simulink model "IP"  (Simulink 5.0)
settings: Solver=ode5  SolverMode=SingleTasking  StartTime=0.0  StopTime=inf  FixedStep=0.001  RelTol=1e-3
libraries: pci1711 x3
settings Model: LastModifiedBy=AD  ExtModeMexFile=rtwinext  SimulationMode=external  TimeSaveName=t  OutputSaveName=y  LimitDataPoints=off  RTWSystemTargetFile=rtwinfbk.tlc  RTWTemplateMakefile=winfbktmf  RTWOptions="-aCCOptimize=1 -aEnforceIntegerDowncast=1 -aExtMode=1 -aFoldNonRolledExpr=1 -aForceParamTrailComments=0 -aGenerateComments=1 -aGenerateReport=0 -aIncDataTypeInIds=0 -aIncHierarchyInIds=0 -aInlineInvariantSignals=0 -aInlineParameters=0 -aInlinedPrmAccess=\"Literals\" -aLocalBlockOutputs=1 -aMaxRTWIdLen=31 -aPrefixModelToSubsysFcnNames=1 -aRTWVerbose=1 -aRebuildAll=0 -aRollThreshold=5 -aShowEliminatedStatements=0"

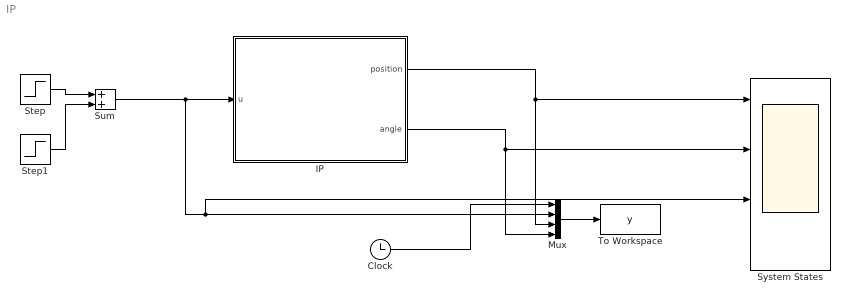
== system IP ==
  Clock : Clock
  IP : Subsystem
  Mux : Mux
  Step : Step  After=0  SampleTime=0
  Step1 : Step  Time=1.4  After=0  SampleTime=0
  Sum : Sum  SaturateOnIntegerOverflow=on
  System States : Scope  NumInputPorts=4
      settings: TimeRange=70  YMin=-0.0025~-0.5~-1~-15  YMax=0.002~3.5~1~15  Decimation=0.1  SampleInput=on  SampleTime=0.01
  To Workspace : ToWorkspace  VariableName=y  SampleTime=0.001  SaveFormat=Array
  wires:
  Step/1 -> Sum/1
  Step1/1 -> Sum/2
  Sum/1 -> IP/1(u), Mux/2, System States/3
  Clock/1 -> Mux/1
  Mux/1 -> To Workspace/1
  IP/1(position) -> Mux/3, System States/1
  IP/2(angle) -> Mux/4, System States/2

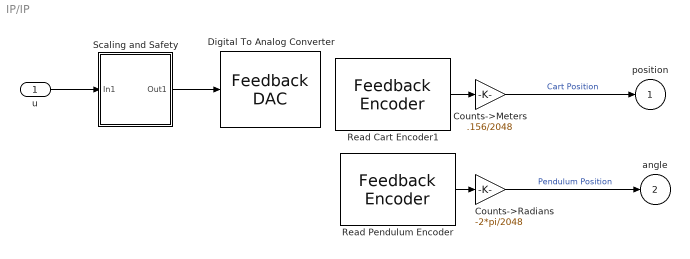
== system IP/IP ==
  u : Inport
  Counts->Meters : Gain  Gain=.156/2048  SaturateOnIntegerOverflow=on
  Counts->Radians : Gain  Gain=-2*pi/2048  SaturateOnIntegerOverflow=on
  Digital To Analog Converter : pci1711/Advantech  PCI1711 I//O Board Lib/Feedback DAC  channel=0  range=0  tsamp=0.001  hwAccess=on
  Read Cart Encoder1 : pci1711/Advantech  PCI1711 I//O Board Lib/Feedback Encoder   channel=0  offset=0  tsamp=0.001  hwAccess=on
  Read Pendulum Encoder : pci1711/Advantech  PCI1711 I//O Board Lib/Feedback Encoder   channel=1  offset=-1024  tsamp=0.001  hwAccess=on
  Scaling and Safety : Subsystem
  position : Outport
  angle : Outport  Port=2
  wires:
  Counts->Meters/1 -> position/1  "Cart Position"
  Counts->Radians/1 -> angle/1  "Pendulum Position"
  Read Pendulum Encoder/1 -> Counts->Radians/1
  Read Cart Encoder1/1 -> Counts->Meters/1
  u/1 -> Scaling and Safety/1(In1)
  Scaling and Safety/1(Out1) -> Digital To Analog Converter/1

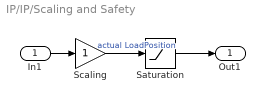
== system IP/IP/Scaling and Safety ==
  In1 : Inport
  Saturation : Saturate  UpperLimit=2.5  LowerLimit=-2.5
  Scaling : Gain  SaturateOnIntegerOverflow=on
  Out1 : Outport
  wires:
  Saturation/1 -> Out1/1
  In1/1 -> Scaling/1
  Scaling/1 -> Saturation/1  "actual LoadPosition"
